simulink model "Suspension_model"  (R2020b)
settings: Solver=VariableStepAuto  StartTime=0.0  StopTime=60  RelTol=1e-3
undefined symbols (not defined in the file or in its folder): B, K1, K2, M1, M2
settings Model: DataDictionary=model_data.sldd  EnableAccessToBaseWorkspace=off  Creator=153  LastModifiedBy=153

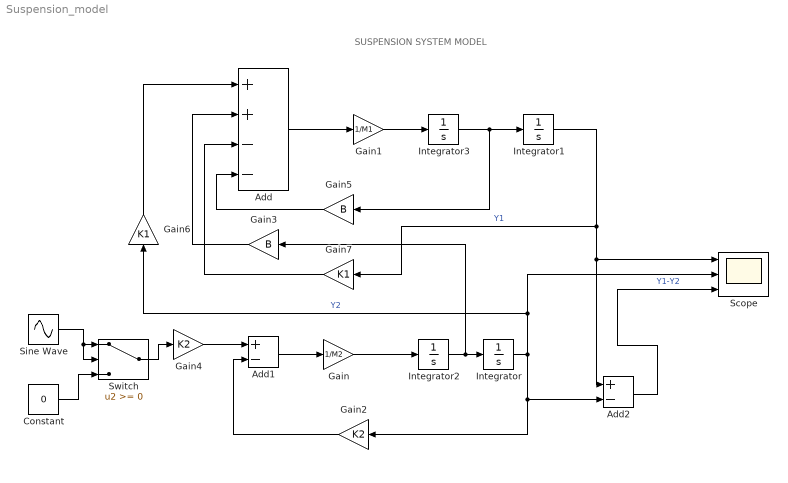
== system Suspension_model ==
  note: SUSPENSION SYSTEM MODEL
  Add : Sum  Inputs=++--
  Add1 : Sum  Inputs=+-
  Add2 : Sum  Inputs=+-
  Constant : Constant  Value=0
  Gain : Gain  Gain=1/M2
  Gain1 : Gain  Gain=1/M1
  Gain2 : Gain  Gain=K2
  Gain3 : Gain  Gain=B
  Gain4 : Gain  Gain=K2
  Gain5 : Gain  Gain=B
  Gain6 : Gain  Gain=K1
  Gain7 : Gain  Gain=K1
  Integrator{,1..3} (4 alike) : Integrator
  Scope : Scope  NumInputPorts=3
  Sine Wave : Sin  SampleTime=0
  Switch : Switch
  wires:
  Gain4/1 -> Add1/1
  Add1/1 -> Gain/1
  Gain/1 -> Integrator2/1
  Integrator/1 -> Scope/2, Gain6/1, Add2/2, Gain2/1  "Y2"
  Gain2/1 -> Add1/2
  Gain5/1 -> Add/4
  Gain1/1 -> Integrator3/1
  Add/1 -> Gain1/1
  Integrator2/1 -> Gain3/1, Integrator/1
  Integrator3/1 -> Gain5/1, Integrator1/1
  Integrator1/1 -> Add2/1, Scope/1, Gain7/1  "Y1"
  Gain3/1 -> Add/2
  Gain7/1 -> Add/3
  Gain6/1 -> Add/1
  Sine Wave/1 -> Switch/2, Switch/1
  Constant/1 -> Switch/3
  Switch/1 -> Gain4/1
  Add2/1 -> Scope/3  "Y1-Y2"
